simulink model "motorsim"  (R2018a)
settings: Solver=FixedStepAuto  StartTime=0.0  StopTime=3  FixedStep=1/30e3  RelTol=1e-3  EnableMultiTasking=on
undefined symbols (not defined in the file): MotorParams, MtrCtrlMd, sigbuilder_block
settings Model: PauseTimes=0.1  Creator=uids8840  LastModifiedBy=elrobotista
settings SolverCC: AlgebraicLoopSolver=LineSearch
settings DataIOCC: LimitDataPoints=on  SaveFormat=Array  SaveOutput=off  DSMLogging=off  SaveTime=off
settings OptimizationCC: DefaultParameterBehavior=Inlined  UseFloatMulNetSlope=on  DefaultUnderspecifiedDataType=single  InlineInvariantSignals=on  PassReuseOutputArgsAs=Individual arguments  ZeroExternalMemoryAtStartup=off  ZeroInternalMemoryAtStartup=off  NoFixptDivByZeroProtection=on  EfficientFloat2IntCast=on  LifeSpan=1
settings DebuggingCC: SolverPrmCheckMsg=warning  MultiTaskRateTransMsg=warning  ParameterTunabilityLossMsg=error  SFUnexpectedBacktrackingDiag=warning  SFNoUnconditionalDefaultTransitionDiag=warning  SFExecutionAtInitializationDiag=none
settings HardwareCC: ProdBitPerPointer=32  ProdBitPerSizeT=32  ProdBitPerPtrDiffT=32  ProdLargestAtomicInteger=Long  ProdLargestAtomicFloat=Double  ProdWordSize=32  ProdHWDeviceType=ARM Compatible->ARM Cortex
settings ModelReferenceCC: UpdateModelReferenceTargets=IfOutOfDate  EnableRefExpFcnMdlSchedulingChecks=off  ModelReferenceNumInstancesAllowed=Single  PropagateSignalLabelsOutOfModel=off
settings SFSimCC: SFSimEcho=off  SimCtrlC=off  SimIntegrity=off  MATLABDynamicMemAlloc=off
settings RTWCC: SystemTargetFile=ert.tlc  TemplateMakefile=ert_default_tmf  GenerateReport=on  IncludeHyperlinkInReport=on  LaunchReport=on  GenerateTraceInfo=on  GenerateTraceReport=on  GenerateTraceReportSl=on  GenerateTraceReportSf=on  GenerateTraceReportEml=on  GenerateCodeMetricsReport=on
settings CodeAppCC: ForceParamTrailComments=on  IgnoreCustomStorageClasses=off  OperatorAnnotations=on  SimulinkDataObjDesc=on  SFDataObjDesc=on  CustomSymbolStrGlobalVar=rt$N$M  CustomSymbolStrType=$N$M  CustomSymbolStrFcn=$N$M$F  CustomSymbolStrMacro=$N$M  InsertBlockDesc=on  StateflowObjectComments=on
settings ERTTargetCC: GenerateSampleERTMain=on  IncludeMdlTerminateFcn=off  CombineSignalStateStructs=on  SupportComplex=off  InlinedParameterPlacement=NonHierarchical  ERTCustomFileTemplate=example_file_process.tlc
settings ConfigComp: CovMetricSettings=dw  CovHtmlReporting=on  CovSaveCumulativeToWorkspaceVar=on  CovSaveSingleToWorkspaceVar=on  CovExternalEMLEnable=off

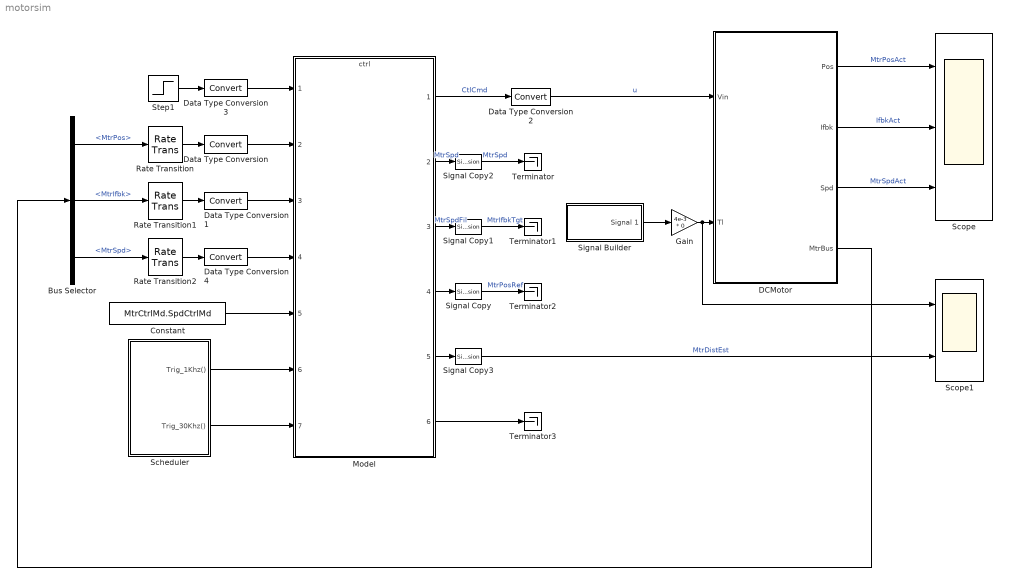
== system motorsim ==
  Bus Selector : BusSelector  OutputSignals=MtrPos,MtrIfbk,MtrSpd
  Constant : Constant  Value=MtrCtrlMd.SpdCtrlMd
  DCMotor : Subsystem
  Data Type Conversion{,1..4} (5 alike) : DataTypeConversion
  Gain : Gain  Gain=4e-3 * 0
  Model : ModelReference  ModelNameDialog=ctrl  SimulationMode=Normal  ModelReferenceVersion=1.654
  Rate Transition : RateTransition
  Rate Transition1 : RateTransition
  Rate Transition2 : RateTransition
  Scheduler : Stateflow chart  TreatAsAtomicUnit=on  SystemSampleTime=1/30e3
  Scope : Scope  NumInputPorts=3
  Scope1 : Scope  NumInputPorts=2
  Signal Builder : Subsystem  Tag=STV Subsys  LoadFcn=sigbuilder_block('load');  StartFcn=sigbuilder_block('start');  StopFcn=sigbuilder_block('stop');  ClipboardFcn=sigbuilder_block('clipboard');  mask(Sigbuilder block){tuvar=[0:10]}
      mask help: Simulink:masks:SigbuilderBlock_MD
      mask init:
      | if ~strcmp(get_param(bdroot(gcbh),'SimulationStatus'),'stopped') tuvar = sigbuilder_block('maskInit'); end
      settings: CopyFcn=sigbuilder_block('copy');  DeleteFcn=sigbuilder_block('delete');  ModelCloseFcn=sigbuilder_block('modelClose');  PreSaveFcn=sigbuilder_block('preSave');  PauseFcn=sigbuilder_block('pause');  ContinueFcn=sigbuilder_block('continue');  NameChangeFcn=sigbuilder_block('namechange');  OpenFcn=sigbuilder_block('open',[437.25 199.5 550.5 399.75 ]);  CloseFcn=sigbuilder_block('close');
      mask Display: plot(0, 0, 100, 100,[2, 2, 32, 32, 2], [68, 8, 8, 68, 68],[32, 2], [38, 38], [32, 19, 2],[53, 60, 44], [32, 17, 17, 2],[16, 16, 31, 31]);txt = getActiveGroup(gcbh);text(2, 100, txt,'verticalAlignment', 'top');
  Signal Copy{,1..3} (4 alike) : SignalConversion  OverrideOpt=off
  Step1 : Step  Time=0  After=500  SampleTime=0
  Terminator{,1..3} (4 alike) : Terminator
  wires:
  Constant/1 -> Model/5
  Scheduler/1(Trig_1Khz()) -> Model/6
  Model/1 -> Data Type Conversion2/1  "CtlCmd"
  Scheduler/2(Trig_30Khz()) -> Model/7
  Model/2 -> Signal Copy2/1  "MtrSpd"
  Model/3 -> Signal Copy1/1  "MtrSpdFil"
  Model/4 -> Signal Copy/1
  Model/5 -> Signal Copy3/1
  Step1/1 -> Data Type Conversion3/1
  DCMotor/4(MtrBus) -> Bus Selector/1
  Data Type Conversion/1 -> Model/2
  Data Type Conversion3/1 -> Model/1
  DCMotor/3(Spd) -> Scope/3  "MtrSpdAct"
  DCMotor/2(Ifbk) -> Scope/2  "IfbkAct"
  DCMotor/1(Pos) -> Scope/1  "MtrPosAct"
  Signal Copy/1 -> Terminator2/1  "MtrPosRef"
  Rate Transition/1 -> Data Type Conversion/1
  Rate Transition1/1 -> Data Type Conversion1/1
  Signal Copy1/1 -> Terminator1/1  "MtrIfbkTgt"
  Signal Copy2/1 -> Terminator/1  "MtrSpd"
  Rate Transition2/1 -> Data Type Conversion4/1
  Data Type Conversion4/1 -> Model/4
  Bus Selector/3 -> Rate Transition2/1  "<MtrSpd>"
  Bus Selector/2 -> Rate Transition1/1  "<MtrIfbk>"
  Bus Selector/1 -> Rate Transition/1  "<MtrPos>"
  Data Type Conversion2/1 -> DCMotor/1(Vin)  "u"
  Signal Builder/1(Signal 1) -> Gain/1
  Gain/1 -> Scope1/1, DCMotor/2(Tl)
  Model/6 -> Terminator3/1
  Signal Copy3/1 -> Scope1/2  "MtrDistEst"
  Data Type Conversion1/1 -> Model/3

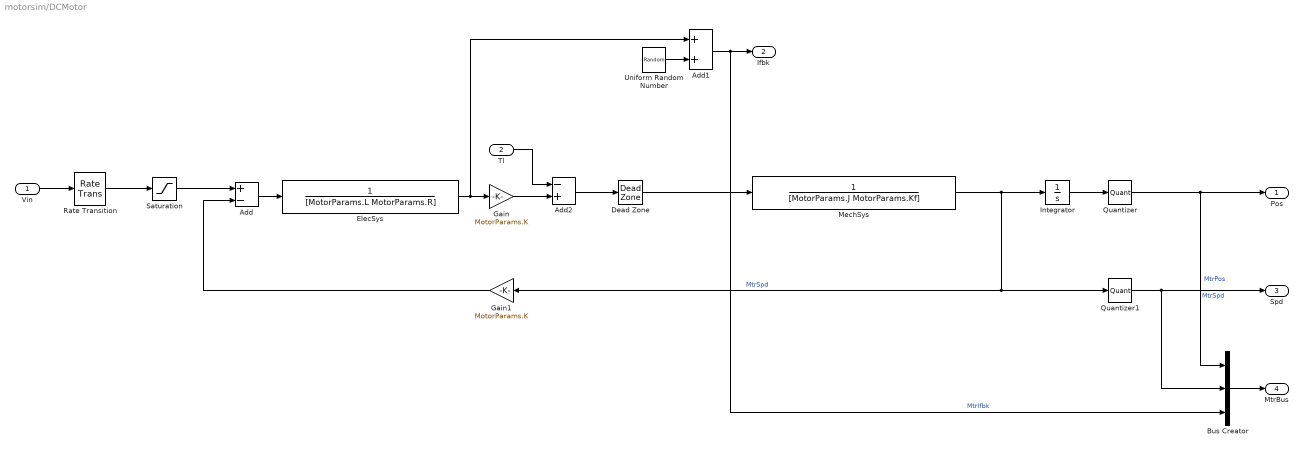
== system motorsim/DCMotor ==
  Vin : Inport
  Tl : Inport  Port=2
  Add : Sum  Inputs=+-
  Add1 : Sum
  Add2 : Sum  Inputs=-+
  Bus Creator : BusCreator  Inputs=3
  Dead Zone : DeadZone  LowerValue=-7.7e-4  UpperValue=7.7e-4  SaturateOnIntegerOverflow=on
      settings: AttributesFormatString=[%<LowerValue>, %<UpperValue>]
  ElecSys : TransferFcn  Denominator=[MotorParams.L MotorParams.R]
  Gain : Gain  Gain=MotorParams.K
      settings: AttributesFormatString=%<Gain>
  Gain1 : Gain  Gain=MotorParams.K
      settings: AttributesFormatString=%<Gain>
  Integrator : Integrator
  MechSys : TransferFcn  Denominator=[MotorParams.J MotorParams.Kf]
  Quantizer : Quantizer  QuantizationInterval=2*pi/4000
  Quantizer1 : Quantizer  QuantizationInterval=2*pi/4000
  Rate Transition : RateTransition
  Saturation : Saturate  UpperLimit=12  LowerLimit=-12
      settings: AttributesFormatString=[%<LowerLimit>, %<UpperLimit>]
  Uniform Random Number : UniformRandomNumber  Minimum=-10e-3  Maximum=10e-3
  Pos : Outport
  Ifbk : Outport  Port=2
  Spd : Outport  Port=3
  MtrBus : Outport  Port=4
  wires:
  Add/1 -> ElecSys/1
  ElecSys/1 -> Gain/1, Add1/1
  Gain/1 -> Add2/2
  Add1/1 -> Bus Creator/3, Ifbk/1  "MtrIfbk"
  Uniform Random Number/1 -> Add1/2
  Gain1/1 -> Add/2
  Vin/1 -> Rate Transition/1
  MechSys/1 -> Integrator/1, Quantizer1/1, Gain1/1  "MtrSpd"
  Saturation/1 -> Add/1
  Tl/1 -> Add2/1
  Bus Creator/1 -> MtrBus/1
  Integrator/1 -> Quantizer/1
  Rate Transition/1 -> Saturation/1
  Quantizer/1 -> Pos/1, Bus Creator/1  "MtrPos"
  Quantizer1/1 -> Bus Creator/2, Spd/1  "MtrSpd"
  Dead Zone/1 -> MechSys/1
  Add2/1 -> Dead Zone/1

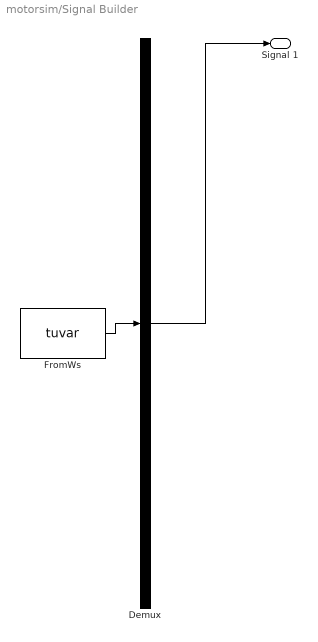
== system motorsim/Signal Builder ==
  Demux : Demux  Tag=STV Demux  Outputs=1
  FromWs : FromWorkspace  Tag=STV FromWs  VariableName=tuvar  SampleTime=0
      SigBuilderData=|
      | common.afterFinalStr = 'Extrapolate'
      | common.sampleTime = 0
      | dataSet.timeRange = [0 3]
      | dataSet.name = 'Group 1'
      | sbobj.Groups.Name = 'Group 1'
      | sbobj.Groups.Signals.Name = 'Signal 1'
      | sbobj.Groups.Signals.XData = [0 0.225 0.555 1.165 2.36 3]
      | sbobj.Groups.Signals.YData = [0 0 0.945 -0.27 0.275 0.06]
      | sbobj.Groups.TimeRange = [0 3]
  Signal 1 : Outport  Tag=STV Outport
  wires:
  Demux/1 -> Signal 1/1
  FromWs/1 -> Demux/1

== stateflow chart motorsim/Scheduler ==
  (default) -> (junction 26)
  (junction 26) -> (junction 25) [order 1] : [cnt == 0]
  (junction 25) -> (junction 1)
  (junction 26) -> (junction 1) [order 2]
  (junction 1) -> (junction 15) [order 1] : [!(cnt %% TASK_COUNT_30KHZ)]{Trig_30Khz;}
  (junction 15) -> (junction 9)
  (junction 1) -> (junction 9) [order 2]
  (junction 9) -> (junction 18) [order 1] : [!(cnt %% TASK_COUNT_1KHZ)] {Trig_1Khz;}
  (junction 18) -> (junction 19) : {cnt = 1;}
  (junction 9) -> (junction 19) [order 2] : {cnt++;}
  data: TASK_COUNT_1KHZ constant uint32 size=1 =30; TASK_COUNT_30KHZ constant uint32 size=1 =1; cnt local uint32 size=1 =0; F_RATE local uint32 size=1 =30e3; dbg_out local double
  events: Trig_1Khz output FUNCTION_CALL_EVENT; Trig_30Khz output FUNCTION_CALL_EVENT
